simulink model "SimulationWorking"  (R2016b)
settings: Solver=FixedStepDiscrete  StartTime=0.0  StopTime=1  RelTol=1e-3  EnableMultiTasking=on
libraries: commdigbbndpm3 x3, commrflib2 x2, commrfcorlib x1, commutil2 x1
settings Model: Creator=Lab  LastModifiedBy=Rickard
settings SolverCC: ConcurrentTasks=on  AutoInsertRateTranBlk=on  InsertRTBMode=Always
settings DataIOCC: SaveFormat=StructureWithTime
settings OptimizationCC: BlockReduction=off  OptimizeBlockIOStorage=off  BufferReuse=off  GlobalBufferReuse=off  ExpressionFolding=off  PassReuseOutputArgsAs=Individual arguments  LocalBlockOutputs=off
settings DebuggingCC: ParameterTunabilityLossMsg=error
settings HardwareCC: ProdBitPerInt=16  ProdBitPerPointer=16  ProdBitPerSizeT=16  ProdBitPerPtrDiffT=16  ProdLargestAtomicFloat=None  ProdWordSize=8  ProdHWDeviceType=Atmel->AVR
settings RTWCC: SystemTargetFile=realtime.tlc  GenerateMakefile=off  TemplateMakefile=realtime.tmf  Description=Run on Target Hardware  GenerateReport=on  RTWVerbose=off  IncludeHyperlinkInReport=on  LaunchReport=on  CodeExecutionProfiling=on  GenerateTraceInfo=on  GenerateTraceReport=on  GenerateTraceReportSl=on  GenerateTraceReportSf=on  GenerateTraceReportEml=on  RTWCompilerOptimization=on
settings CodeAppCC: ForceParamTrailComments=on  IgnoreCustomStorageClasses=off  OperatorAnnotations=on  SimulinkDataObjDesc=on  SFDataObjDesc=on  InsertBlockDesc=on
settings STFCustomTargetCC: TargetLibSuffix=.a  MultiwordLength=256  GenerateSampleERTMain=on  CombineOutputUpdateFcns=on  ERTCustomFileBanners=on  SupportContinuousTime=off  SupportNonInlinedSFcns=off  RemoveResetFunc=on  MATLABClassNameForMDSCustomization=Simulink.SoftwareTarget.ERTCustomization  GRTInterface=off  SystemTargetFile=realtime.tlc
settings ERTTargetCC: MultiwordLength=256  GenerateSampleERTMain=on  ParMdlRefBuildCompliant=off  CompOptLevelCompliant=off  ConcurrentExecutionCompliant=off  ERTFirstTimeCompliant=off  ModelStepFunctionPrototypeControlCompliant=off  CPPClassGenCompliant=off  UseToolchainInfoCompliant=off  ERTCustomFileTemplate=realtime_file_process.tlc

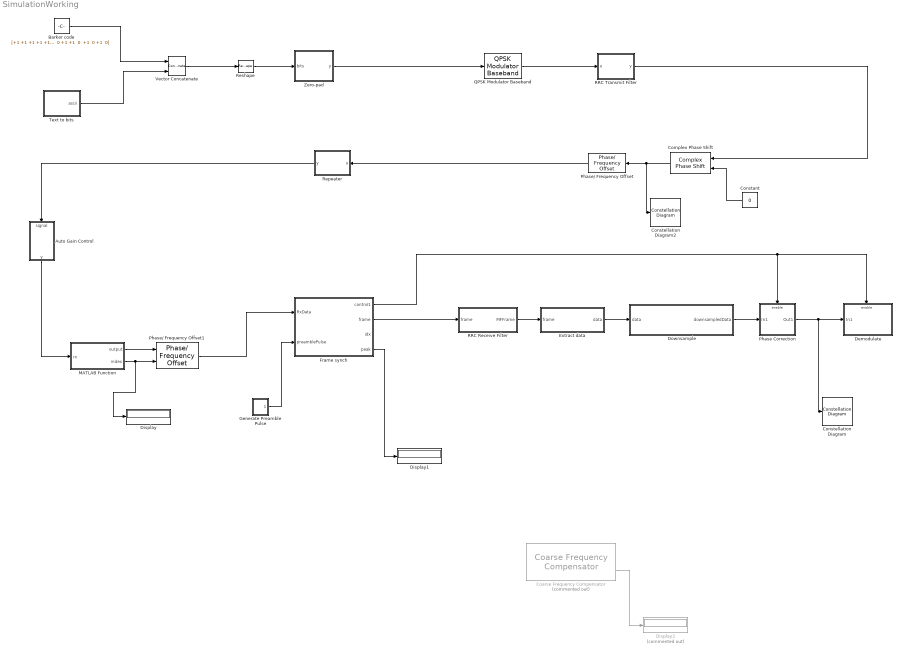
== system SimulationWorking ==
  Auto Gain Control : MATLAB Function  TreatAsAtomicUnit=on
  Barker code : Constant  Value="[+1 +1 +1 +1 +1 0  0 +1 +1  0  +1  0 +1  0 +1 +1 +1 +1 +1 0  0 +1 +1  0  +1  0 +1  0]"  VectorParams1D=off  SampleTime=-1
  Coarse Frequency Compensator : commrfcorlib/Coarse Frequency Compensator  Commented=on  Modulation=QPSK  Algorithm=FFT-based  FrequencyResolution=0.1  MaximumFrequencyOffset=1  EstimatedFreqOffsetPort=on  SimulateUsing=Code generation
  Complex Phase Shift : commutil2/Complex Phase Shift
  Constant : Constant  Value=0
  Constellation Diagram : ConstellationDiagram
  Constellation Diagram2 : ConstellationDiagram
  "Demodulate " : Subsystem
  Display : Display
  Display1 : Display
  Display2 : Display  Commented=on
  Downsample : MATLAB Function  TreatAsAtomicUnit=on
  Extract data : MATLAB Function  TreatAsAtomicUnit=on
  "Frame synch " : MATLAB Function  TreatAsAtomicUnit=on
  "Generate Preamble Pulse " : Subsystem
  MATLAB Function : MATLAB Function  TreatAsAtomicUnit=on
  Phase Correction : Subsystem
  Phase/ Frequency Offset : commrflib2/Phase// Frequency Offset  phaseOffset=0  freqPort=off  freqOffset=300
  Phase/ Frequency Offset1 : commrflib2/Phase// Frequency Offset  phaseOffset=0  freqPort=on  freqOffset=-200
  QPSK Modulator Baseband : commdigbbndpm3/QPSK Modulator Baseband  InType=Bit  Enc=Gray  Ph=pi/4  outDtype=double  outWordLen=16  outUDDataType=sfix(16)  outFracLenMode=Best precision  outFracLen=15  outDataTypeStr=double  outLastDataTypeStr=double
  RRC Receive Filter : MATLAB Function  TreatAsAtomicUnit=on
  RRC Transmit Filter : MATLAB Function  TreatAsAtomicUnit=on
  Repeater : MATLAB Function  TreatAsAtomicUnit=on
  Reshape : Reshape  OutputDimensionality=Column vector (2-D)
  "Text to bits " : MATLAB Function  TreatAsAtomicUnit=on
  Vector Concatenate : Concatenate
  "Zero-pad " : MATLAB Function  TreatAsAtomicUnit=on
  wires:
  Reshape/1 -> "Zero-pad "/1(bits)
  "Text to bits "/1(ascii) -> Vector Concatenate/2
  Vector Concatenate/1 -> Reshape/1
  "Zero-pad "/1(y) -> QPSK Modulator Baseband/1
  Barker code/1 -> Vector Concatenate/1
  QPSK Modulator Baseband/1 -> RRC Transmit Filter/1(u)
  RRC Receive Filter/1(MFFrame) -> Extract data/1(frame)
  "Frame synch "/2(frame) -> RRC Receive Filter/1(frame)
  Extract data/1(data) -> Downsample/1(data)
  Downsample/1(downsampledData) -> Phase Correction/1(In1)
  Phase Correction/1(Out1) -> "Demodulate "/1(In1), Constellation Diagram/1
  "Frame synch "/1(control1) -> Phase Correction/Enable, "Demodulate "/Enable
  Phase/ Frequency Offset/1 -> Repeater/1(u)
  "Frame synch "/4(peak) -> Display1/1
  MATLAB Function/1(output) -> Phase/ Frequency Offset1/1
  MATLAB Function/2(index) -> Display/1, Phase/ Frequency Offset1/2
  RRC Transmit Filter/1(y) -> Complex Phase Shift/1
  Complex Phase Shift/1 -> Constellation Diagram2/1, Phase/ Frequency Offset/1
  Constant/1 -> Complex Phase Shift/2
  Coarse Frequency Compensator/2 -> Display2/1
  Auto Gain Control/1(y) -> MATLAB Function/1(rx)
  Phase/ Frequency Offset1/1 -> "Frame synch "/1(RxData)
  "Generate Preamble Pulse "/1(Out1) -> "Frame synch "/2(preamblePulse)
  Repeater/1(y) -> Auto Gain Control/1(signal)

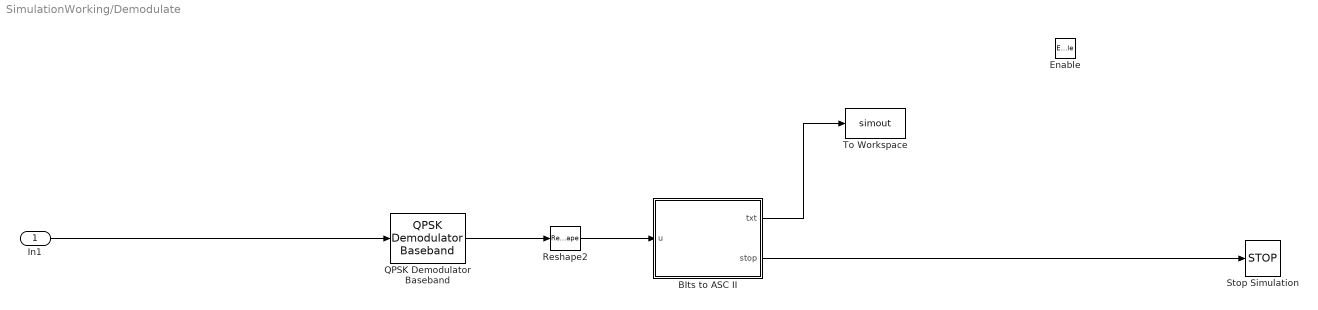
== system SimulationWorking/Demodulate  ==
  In1 : Inport
  Enable : EnablePort  StatesWhenEnabling=reset  PropagateVarSize=During execution
  BIts to ASC II : MATLAB Function  TreatAsAtomicUnit=on
  QPSK Demodulator Baseband : commdigbbndpm3/QPSK Demodulator Baseband  OutType=Bit  DecType=Hard decision  VarSource=Dialog  Variance=1  Dec=Gray  Ph=pi/4  outDtype1=Inherit via internal rule  outDtype2=Inherit via internal rule  derotateFactorWordLen=16  derotateFactorDataTypeStr=Inherit: Same word length as input  derotateFactorLastDataTypeStr=Inherit: Same word length as input
  Reshape2 : Reshape  OutputDimensionality=Row vector (2-D)
  Stop Simulation : Stop
  To Workspace : ToWorkspace  VariableName=simout  SaveFormat=Structure  SampleTime=-1
  wires:
  In1/1 -> QPSK Demodulator Baseband/1
  Reshape2/1 -> BIts to ASC II/1(u)
  QPSK Demodulator Baseband/1 -> Reshape2/1
  BIts to ASC II/1(txt) -> To Workspace/1
  BIts to ASC II/2(stop) -> Stop Simulation/1

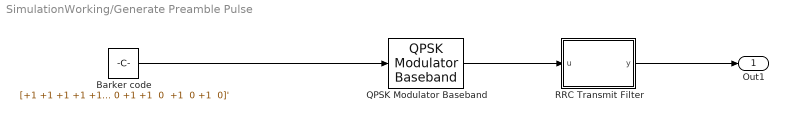
== system SimulationWorking/Generate Preamble Pulse  ==
  Barker code : Constant  Value="[+1 +1 +1 +1 +1 0  0 +1 +1  0  +1  0 +1  0 +1 +1 +1 +1 +1 0  0 +1 +1  0  +1  0 +1  0]'"  VectorParams1D=off  SampleTime=-1
  QPSK Modulator Baseband : commdigbbndpm3/QPSK Modulator Baseband  InType=Bit  Enc=Gray  Ph=pi/4  outDtype=double  outWordLen=16  outUDDataType=sfix(16)  outFracLenMode=Best precision  outFracLen=15  outDataTypeStr=double  outLastDataTypeStr=double
  RRC Transmit Filter : MATLAB Function  TreatAsAtomicUnit=on
  Out1 : Outport
  wires:
  QPSK Modulator Baseband/1 -> RRC Transmit Filter/1(u)
  Barker code/1 -> QPSK Modulator Baseband/1
  RRC Transmit Filter/1(y) -> Out1/1

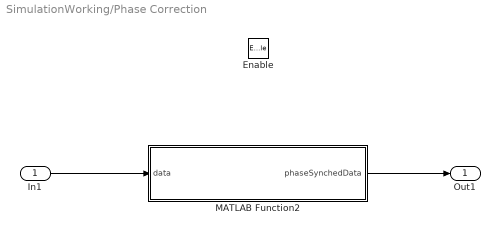
== system SimulationWorking/Phase Correction ==
  In1 : Inport
  Enable : EnablePort  StatesWhenEnabling=reset  PropagateVarSize=During execution
  MATLAB Function2 : MATLAB Function  TreatAsAtomicUnit=on
  Out1 : Outport
  wires:
  MATLAB Function2/1(phaseSynchedData) -> Out1/1
  In1/1 -> MATLAB Function2/1(data)

== matlab function SimulationWorking/Repeater ==
  data: u input; y output
function y = fcn(u)

y = repmat(u',1,2)';

== matlab function SimulationWorking/Text to bits  ==
  data: ascii output

function ascii = fcn
    frame_length = 100; 
    txt = 'Hello World #0 Hello World #1 Hello World #2 Hello World #3';
    str = char(zeros(1, frame_length));
    
    % Pad message with char(1)'s to make the frame 100 long
    if length(txt) < frame_length 
        pad = 42*ones(1,frame_length-length(txt));
%         pad = randi([100 250], 1, frame_length-length(txt)); 
        tmp = double(txt); 
        tmp1 = [tmp pad]; 
        str = char(tmp1); 
        
    end
    
    
    
    symbols = zeros(1, length(str));
    bits =  zeros(length(str), 8); 
    ascii = zeros(1,8*length(str)); 
    
    
     
    
    symbols = double(char(str));
    bits = de2bi(symbols, 'left-msb', 8);
    
   
    ascii = reshape(bits', [1 8*size((bits),1)]);
    
    %% test with 00 01 10 11
%     txt=[0 0 0 1 1 0 1 1 0 0 0 1 1 0 1 1 0 0 0 1 1 0 1 1 0 0 0 1 1 0 1 1 0 0 0 1 1 0 1 1 0 0 0 1 1 0 1 1];
%        if length(txt) < frame_length 
%         pad = 42*zeros(1,frame_length-length(txt)); 
%         tmp1 = [txt pad]; 
%        end
%    ascii=tmp1;
%        
%         
   
end

== matlab function SimulationWorking/Demodulate /BIts to ASC II ==
  data: u input; txt output double size=[1 100]; stop output
function [txt, stop] = BITS2ASCII(u)


len=floor(length(u)/8);  
asc = ones(1,len);
multi=[128 64 32 16 8 4 2 1];


for i=1:len
 asc_bits=u(:, 8*i-7:8*i);
 ascnum = sum(asc_bits.*multi);
 asc(1,i)= ascnum;
end 
 
txt = asc; 
% Remove *-padding. 
% idx = find(asc==42);
% txt = asc(1:idx(1)-1); 

disp(char(txt))
stop = 1;       % Control signal to stop simulation 




end

== matlab function SimulationWorking/Frame synch  ==
  settings: updateMethod=DISCRETE
  data: control1 output; frame output size=[1696 1]; idx output; RxData input size=[3392,1]; preamblePulse input; peak output
function [control1, frame,idx,peak]  = fcn(RxData, preamblePulse)

sps = 4;                 % Samples per symbol
frame_length = 414;      % Symbols per frame

crosscorr = abs(xcorr(preamblePulse, RxData)); 
[peak, idx] = max(crosscorr);




if peak > 5 && idx < 1800 
    frame = RxData(idx+1:idx+frame_length*sps); 
    control1 = 1; 
else

    frame = zeros(400*sps,1); 
    control1 = -1; 
end

== matlab function SimulationWorking/RRC Transmit Filter ==
  data: u input; y output
function y = RRC(u)

% This function is a modified version of the one given in the text, Program 2.2-2
% a: Roll off/ Excess bandwidth factor
% tau: Symbol time 
% fs: sampling frequency at which the continuous pulse is sampled
% span: Defines width for truncation. Number of tau periods on either side of the peak of the pulse
% The pulse has a one sided bandwidth, BW = (1+alpha)/(2*tau);
% Choose fs > 2*BW
% Use all the provided functions with caution!

BW = 1e6; 
tau = 1/BW; 
fs = 2.1*BW; 
span = 10; 
a = 0.5; 
sps = 4; 



t_positive = eps:(1/fs):span*tau;  % Replace 0 with eps (smallest +ve number MATLAB can produce) to prevent NANs
t = [-fliplr(t_positive(2:end)) t_positive];
tpi = pi/tau; amtpi = tpi*(1-a); aptpi = tpi*(1 + a);
ac = 4*a/tau; at = 16*a^2/tau^2;
pulse = (sin(amtpi*t) + (ac*t).*cos(aptpi*t))./(tpi*t.*(1-at*t.^2));
% norm_factor = sqrt(sum(pulse.^2));
% pulse = pulse/norm_factor; % Normlaize the pulse to have unit energy

symbols = upsample(u, sps); 
y = conv(pulse,symbols); 

end

== matlab function SimulationWorking/Zero-pad  ==
  data: bits input; y output
function y = fcn(bits)
    len = length(bits); 
    a = ceil(len/4);
    padding=zeros(4*a-len, 1);
    
    
    y = zeros(4*a,1); 
    y = [bits; padding]; 
    
      
end

== matlab function SimulationWorking/Extract data ==
  data: frame input size=[1656 1]; data output size=[1600 1]
function data = fcn(frame)

% Preamble is 14 symbols long. Upsampled by 4 --> 56 symbols.
% Extract data only
data = frame(56+1:end);

== matlab function SimulationWorking/Generate Preamble Pulse /RRC Transmit Filter ==
  data: u input; y output
function y = RRC(u)

rolloff = 0.5;        % Roll-off factor
span = 10;           % Truncate (number of symbols)
sps = 4;            % Samples per symbol

txfilter = comm.RaisedCosineTransmitFilter('RolloffFactor',rolloff, ...
    'FilterSpanInSymbols',span,'OutputSamplesPerSymbol',sps);


y = txfilter(u); 

end

== matlab function SimulationWorking/RRC Receive Filter ==
  data: MFFrame output size=[1656 1]; frame input size=[1696,1]
function MFFrame = fcn(frame)
% out = zeros(1600,1); 
% This function is a modified version of the one given in the text, Program 2.2-2
% a: Roll off/ Excess bandwidth factor
% tau: Symbol time 
% fs: sampling frequency at which the continuous pulse is sampled
% span: Defines width for truncation. Number of tau periods on either side of the peak of the pulse
% The pulse has a one sided bandwidth, BW = (1+alpha)/(2*tau);
% Choose fs > 2*BW
% Use all the provided functions with caution!

BW = 1e6; 
tau = 1/BW; 
fs = 2.1*BW; 
span = 10; 
a = 0.5; 





t_positive = eps:(1/fs):span*tau;  % Replace 0 with eps (smallest +ve number MATLAB can produce) to prevent NANs
t = [-fliplr(t_positive(2:end)) t_positive];
tpi = pi/tau; amtpi = tpi*(1-a); aptpi = tpi*(1 + a);
ac = 4*a/tau; at = 16*a^2/tau^2;
pulse = (sin(amtpi*t) + (ac*t).*cos(aptpi*t))./(tpi*t.*(1-at*t.^2));
norm_factor = sqrt(sum(pulse.^2));
pulse = pulse/norm_factor; % Normlaize the pulse to have unit energy

% Matched filter data and down-sample
MF = fliplr(conj(pulse));                             % Matched filter
MF_output = conv(frame,MF);               
MFFrame = MF_output(length(MF):end-length(MF)+1);     % Remove transients



end

== matlab function SimulationWorking/Downsample ==
  settings: sampleTime=1/1.2e6
  data: data input; downsampledData output size=[400 1]
function downsampledData = fcn(data)


sps = 4 ; %downsample factor

% downsampledData = complex(zeros(length(data)/sps, 1));
% tmp = complex(zeros(sps, length(data)/sps));


tmp = reshape(data, [sps length(data)/sps]);
downsampledData = conj(max((tmp)))';




end

== matlab function SimulationWorking/MATLAB Function ==
  data: rx input; output output; index output
function [output,index]= fcompostion(rx)

m = 4;        %modulation order
fsamp =1e6;   %current sample frequency
fr = 10;      %desired resolution
N=2^nextpow2(fsamp/fr); %FFT required points

% SamplesPerSymbol = 4;
% symbolRate = fsamp/SamplesPerSymbol;  %symbol rate

% coef = fsamp/(N*m);
% sigLength = length(rx);
%%
raisedSignal = rx.^m;% Raise the input signal to the M'th power
%% do fft then shift it
absFFTSig = abs(fft(raisedSignal,N));
spectrum = fftshift(absFFTSig);

%%  CALCULATE FREQUENCY OFFSET
% df = fsamp/N;                  % sampling frequency is split into N bins
% fvec = df*(-floor(N/2):1:ceil(N/2)-1); % Truncated, has wide bandwidth
[~, maxIdx] = max(spectrum);

offsetIdx = maxIdx - N/2; 
deltaFreq = fsamp / N; 
index = deltaFreq * (offsetIdx-1) / m; 

% freq = fvec(maxIdx);



index = -(index-200)/10;
output=rx; 




end

== matlab function SimulationWorking/Phase Correction/MATLAB Function2 ==
  data: data input size=[400 1]; phaseSynchedData output size=[400 1]
function phaseSynchedData = phaseSynch(data)

% Correcting phase
a = 0;
mu = 0.01; 

for i = 1:length(data)
       ang = angle(data(i)) + a; 
       ang_correct = floor(ang*2/pi)*pi/2+pi/4; 
       e = ang_correct-ang; 
       a = a + mu*e;
       
    
end

phaseSynchedData = data .* exp(1i*(a)); 



disp(a)


end

== matlab function SimulationWorking/Auto Gain Control ==
  data: signal input; y output
function y = AGC(signal)
    N = length(signal);   % Length of signal
    upsample = 4; 
    Pout = 10*log10(1/upsample);   % Desired output in dB
    
    
    Pout_normal = 10.^(Pout/10); 
    E_normal = sum(abs(signal).^2); 
    
    coef = sqrt(Pout_normal*N/E_normal); 
    y = signal *coef; 
end
